simulink model "NarmaMotorNoDisrtubS2"  (R2019b)
settings: Solver=FixedStepAuto  StartTime=0.0  StopTime=30  FixedStep=0.001  RelTol=1e-3
libraries: neural x1, simulink x1
settings Model: Creator=Emanuel  LastModifiedBy=Emanuel

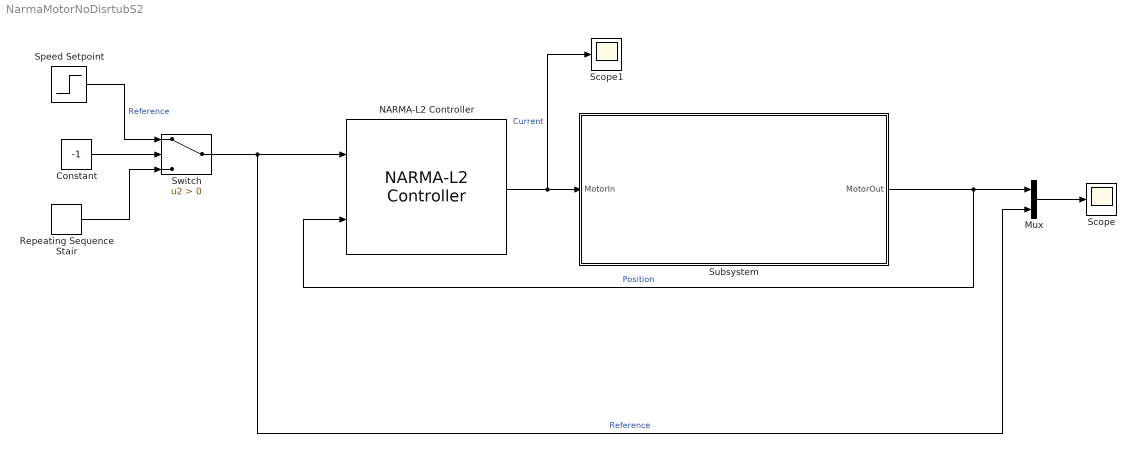
== system NarmaMotorNoDisrtubS2 ==
  Constant : Constant  Value=-1
  Mux : Mux  Inputs=2
  NARMA-L2 Controller : neural/Control Systems/NARMA-L2 Controller  Normalize=0  IW1_1=[-2.974276009383301389 -7.3369230181230387089 -2.9702809109209642457 5.4207339599484667403 7.6507322251574825245 -0.04099227858104749489 -7.6140400707472677411 6.5497336612263019617 4.8034287583779420316 4.8627156977741989863 4.9979580240842551575 12.428056540361712479 10.772508115065093648;-3.7848779205651705837 9.9348214966989338848 18.49827299409104242 -10.090455661305510304 -24.284030478949990339 -5.0384647207874486696 15.653492074662855416 -5.8472817958102094593 -8.3171263007948841306 -4.3483907391506937401 -4.3079358905802287438 -17.852109035411253046 -13.991455106924028939;2.4555196211613341539 -5.4285989222563859613 2.8335778045532187264 -2.2221660495332185015 -18.30929997074996507 0.9608078577356302663 19.398117488478394677 -3.5123739145945203077 -4.2568486454539327113 -5.5331001356038234107 -1.9069745865266656271 -13.104291606894983957 -10.684117094880070553;-15.725226773532602564 11.606034707360642244 -2.4238131705326448895 -10.051560874195246242 7.1499260224029228539 6.8182769946466530442 3.5300431413955801752 -11.667762420868049489 -9.1015914741785337583 -6.0904682598539059413 -14.082250724169222522 2.3580633500480736586 7.6612102121046756764;6.4288402912186972671 9.7333737129299500168 1.5125780634996242036 -4.4898243144994811615 -6.0240011150271524087 -6.203944305279691207 -6.7209811006371422692 9.0984885796634777932 9.6103820236549690748 10.946396320456580398 9.7071762450557628199 14.360221804286766201 13.530671886044359553;-0.00011769746202006098465 1.9131479129218529115e-05 2.1368830884739749535e-06 -2.2538716495860472075e-05 4.4301355498810600407e-05 -1.1306907536450035726e-05 -2.9413442925552235897e-06 -0.0002459300933314099275 0.00014022267822026942869 0.0001254313096875739103 -0.00010130255484437582073 7.0113646745459607193e-05 0.0002621578585166984914;-22.09980172382694974 22.698376943775290471 -14.547253951303501296 -2.1652344301828225781 8.2700319950257590307 5.8782840802360096788 0.47299538496945447985 -1.2446564177901784376 17.92268150488299483 12.162259495231486639 11.853079478572555061 19.970771843250901156 13.138667344604506582]  IW3_2=[1.706627376636813187 2.5735726820080659927 -6.1815669886082655893 0.57275147713232910096 -0.28158305950109818738 -0.40058963532887004177 2.0875189500048016988 -4.5176616794586568204 6.2034230229622489006 0.68314183246592163901 2.7222430817291480842 16.717543720164918852 4.2388903956459351718;10.854169291744398151 4.1599268772786528459 -0.9413361527648951288 -3.4661475675864905632 4.3656951082432797762 3.8319621471641625021 -19.907518954056317995 -13.190558582758342254 -1.7573075764144285849 -6.9276162312328413151 -9.971103171602539561 -18.488983191318666854 -12.655957966149603777;-0.074692547535554681959 0.12448824259257879055 -0.042378075841008985836 -0.0010633351392915922542 -0.047402972676021323806 0.0043997898900478707787 0.025542381717221347703 0.43643985176291932859 -0.040963191110162548714 -0.38753338727414143872 9.0232907589537507675 -4.6628698624088658065 -4.2513664191453219843;3.7161774522690635969 -2.5591393802404667213 -17.714639548587971518 -9.3452325709335468673 12.3521221043333842 18.349937714175496239 18.16388101440478664 -6.5735342650974502021 -1.9388343688512317264 -6.2028994712801530653 -6.9740804318796927319 -15.714806651937312409 -9.0848674503554676107;-0.38561792095397057212 -2.1655339591958520096 3.0795451086940848207 -3.5002169206264666101 -1.5721244517890888837 1.9118640186902990941 2.0413581201640433882 9.9227982049465719427 11.787525530972672527 19.775174712938209609 15.14987346971308213 57.285198652594829127 40.20055653107097271;1.4426181507754287647 -3.2930139520248609131 1.726100971075808399 0.19760804767428463702 -2.7092348185502794777 0.32884589914935780097 2.0362016858337690373 10.354919037811358251 -3.6494508377007615074 12.170550474039952604 1.0545829836571187776 32.166978404432839511 47.464270694044230936;2.1106579591855849642 2.3628910055998768591 -1.7320235272860964315 -1.7164755498128061451 0.21780801521552364819 0.5013567452443652428 -3.2326650559587317701 -0.54820111612144706292 -0.58988404458119769735 -0.18463996511002475631 -0.29562382702827300074 1.3704222651936768251 2.1199608105666714053]  IW5_3=0.042885061780776181917  LW2_1=[-1.7951544843657809558 -0.77607352941402596436 0.028588755459878215787 -0.19678846492423079928 -51.119414104473214877 -178.5855067132064562 -0.066423346363697524652]  LW4_3=[0.63499890113034485051 -1.1080571969744621441 -6.7043348300094498526 3.8041307269777782096 1.5163618754587511184 -1.5268705266003823606 -9.054353426704784269]  LW5_4=3.1544506198367718852  LW6_5=1.8181754716409308514  LW6_2=63.390639269687206081  B1=[0.80241417086431465755;2.1611243877218009324;-1.6799171806335817525;-3.3987486888518860795;-2.9163481938314257391;0.60217891806372336738;-3.2240787265158776798]  B2=53.798959508292931275  B3=[-3.3581424805022304092;-0.021276709706567312891;41.425727380152643775;-0.041722817605074846714;-1.6885845638705636595;-46.221330514506583143;-0.42269984660533566068]  B4=6.1467763144405829223  Limit_output=0  min_output=-Inf  max_output=Inf  Use_Previous_Weights=1  Ts=0.05  S1=7  Ni=7  Nj=7  sim_file=SoleModelNoDistrubance  trainfun=trainlm  Use_validation=1  Use_Testing=1  max_i=40  min_i=1  max_i_int=4  min_i_int=2  sam_training=10000  epochs=500  minp=1.2838861864609374397  maxp=39.753006491435613157  mint=2000.3866487334141766  maxt=39.753006491435613157
      settings: SourceProductName=Deep Learning Toolbox  SourceProductBaseCode=NN
  Repeating Sequence Stair : simulink/Sources/Repeating Sequence Stair  OutValues=[1000 2000 3000 4000 5000].'  tsamp=4  OutMin=[]  OutMax=[]  OutDataTypeStr=double  OutputDataTypeScalingMode=double  OutDataType=fixdt(0,8)  ConRadixGroup=Best Precision: Vector-wise  OutScaling=2^-12
  Scope : Scope
  Scope1 : Scope
  Speed Setpoint : Step  Time=5  Before=2000  After=3000  SampleTime=0
  Subsystem : Subsystem
  Switch : Switch  Criteria=u2 > Threshold
  wires:
  NARMA-L2 Controller/1 -> Scope1/1, Subsystem/1(MotorIn)  "Current"
  Subsystem/1("MotorOut ") -> NARMA-L2 Controller/2, Mux/1  "Position"
  Mux/1 -> Scope/1
  Switch/1 -> Mux/2, NARMA-L2 Controller/1  "Reference"
  Repeating Sequence Stair/1 -> Switch/3
  Speed Setpoint/1 -> Switch/1  "Reference"
  Constant/1 -> Switch/2

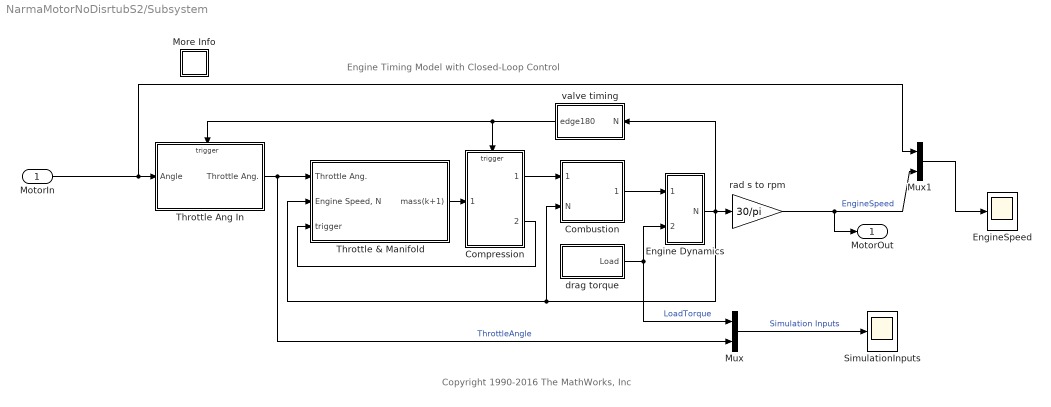
== system NarmaMotorNoDisrtubS2/Subsystem ==
  note: Copyright 1990-2016 The MathWorks, Inc
  note: Engine Timing Model with Closed-Loop Control
  MotorIn : Inport
  Combustion : Subsystem
  Compression : Subsystem  TreatAsAtomicUnit=on
  Engine Dynamics : Subsystem
  EngineSpeed : Scope
  More Info : Subsystem
      settings: OpenFcn=showdemo(bdroot(gcb))
      mask Display: disp('?')
  Mux : Mux  Inputs=2
  Mux1 : Mux  Inputs=2
  SimulationInputs : Scope
  Throttle & Manifold : Subsystem
  Throttle Ang In : Subsystem  TreatAsAtomicUnit=on
  drag torque : Subsystem
  rad s to rpm : Gain  Gain=30/pi  SaturateOnIntegerOverflow=on  OutDataTypeStr=Inherit: Same as input  ParamDataTypeStr=Inherit: Same as input
  valve timing : Subsystem
  "MotorOut " : Outport
  wires:
  Combustion/1(Torque) -> Engine Dynamics/1(Teng)
  Throttle Ang In/1(Throttle Ang.) -> Mux/2, Throttle & Manifold/1(Throttle Ang.)  "ThrottleAngle"
  drag torque/1(Load) -> Mux/1, Engine Dynamics/2(Tload)  "LoadTorque"
  MotorIn/1 -> Mux1/1, Throttle Ang In/1(Angle)
  Throttle & Manifold/1(mass(k+1)) -> Compression/1(mass(k+1))
  Compression/2(trigger) -> Throttle & Manifold/3(trigger)
  Mux/1 -> SimulationInputs/1  "Simulation Inputs"
  rad s to rpm/1 -> "MotorOut "/1, Mux1/2  "EngineSpeed"
  Compression/1(mass(k)) -> Combustion/1(Air Charge)
  Mux1/1 -> EngineSpeed/1
  valve timing/1(edge180) -> Throttle Ang In/Trigger, Compression/Trigger
  Engine Dynamics/1(N) -> rad s to rpm/1, valve timing/1(N), Throttle & Manifold/2("Engine Speed, N"), Combustion/2(N)

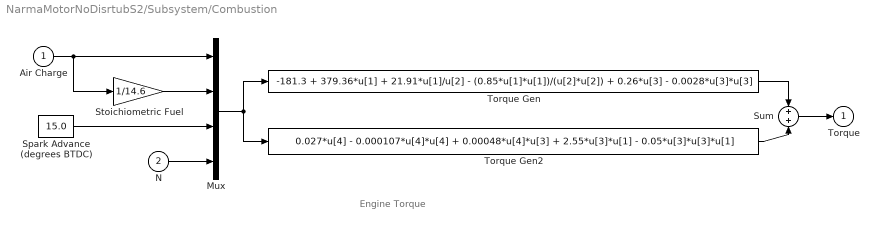
== system NarmaMotorNoDisrtubS2/Subsystem/Combustion ==
  note: Engine Torque
  Air Charge : Inport
  N : Inport  Port=2
  Mux : Mux
  Spark Advance (degrees BTDC) : Constant  Value=15.0
  Stoichiometric Fuel : Gain  Gain=1/14.6  SaturateOnIntegerOverflow=on  OutDataTypeStr=Inherit: Same as input  ParamDataTypeStr=Inherit: Same as input
  Sum : Sum  SaturateOnIntegerOverflow=on  InputSameDT=on  OutDataTypeStr=Inherit: Same as first input
  Torque Gen : Fcn  Expr=-181.3 + 379.36*u[1] + 21.91*u[1]/u[2] - (0.85*u[1]*u[1])/(u[2]*u[2]) + 0.26*u[3] - 0.0028*u[3]*u[3]
  Torque Gen2 : Fcn  Expr=0.027*u[4] - 0.000107*u[4]*u[4] + 0.00048*u[4]*u[3] + 2.55*u[3]*u[1] - 0.05*u[3]*u[3]*u[1]
  Torque : Outport  InitialOutput=0
  wires:
  Stoichiometric Fuel/1 -> Mux/2
  Spark Advance (degrees BTDC)/1 -> Mux/3
  N/1 -> Mux/4
  Air Charge/1 -> Stoichiometric Fuel/1, Mux/1
  Mux/1 -> Torque Gen/1, Torque Gen2/1
  Torque Gen2/1 -> Sum/2
  Torque Gen/1 -> Sum/1
  Sum/1 -> Torque/1

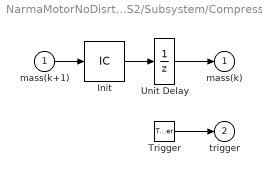
== system NarmaMotorNoDisrtubS2/Subsystem/Compression ==
  mass(k+1) : Inport
  Trigger : TriggerPort  TriggerType=either  VariantControl=Variant  ShowOutputPort=on
  Init : InitialCondition  Value=0.152
  Unit Delay : UnitDelay  InitialCondition=0.152  SampleTime=-1  HasFrameUpgradeWarning=on
  mass(k) : Outport  InitialOutput=0.152
  trigger : Outport  Port=2  InitialOutput=-1
  wires:
  Init/1 -> Unit Delay/1
  mass(k+1)/1 -> Init/1
  Unit Delay/1 -> mass(k)/1
  Trigger/1 -> trigger/1

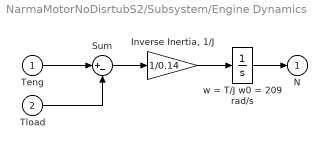
== system NarmaMotorNoDisrtubS2/Subsystem/Engine Dynamics ==
  Teng : Inport
  Tload : Inport  Port=2
  "Inverse Inertia, 1/J" : Gain  Gain=1/0.14  SaturateOnIntegerOverflow=on  OutDataTypeStr=Inherit: Same as input  ParamDataTypeStr=Inherit: Same as input
  Sum : Sum  Inputs=|+-  SaturateOnIntegerOverflow=on  InputSameDT=on  OutDataTypeStr=Inherit: Same as first input
  w = T/J w0 = 209 rad/s : Integrator  InitialCondition=209.48
  N : Outport  InitialOutput=0
  wires:
  "Inverse Inertia, 1/J"/1 -> w = T/J w0 = 209 rad/s/1
  w = T/J w0 = 209 rad/s/1 -> N/1
  Sum/1 -> "Inverse Inertia, 1/J"/1
  Teng/1 -> Sum/1
  Tload/1 -> Sum/2

== system NarmaMotorNoDisrtubS2/Subsystem/More Info ==

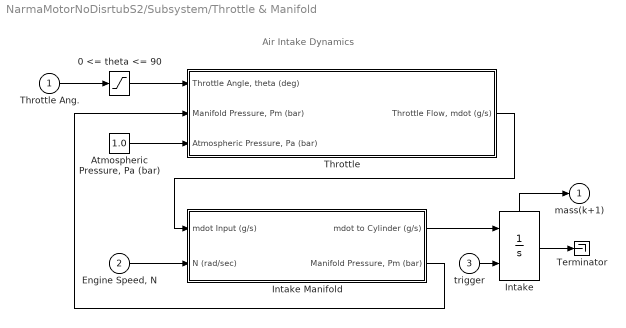
== system NarmaMotorNoDisrtubS2/Subsystem/Throttle & Manifold ==
  note: Air Intake Dynamics
  Throttle Ang. : Inport
  "Engine Speed, N" : Inport  Port=2
  trigger : Inport  Port=3
  0 <= theta <= 90 : Saturate  UpperLimit=90  LowerLimit=0
  "Atmospheric Pressure, Pa (bar)" : Constant  Value=1.0
  Intake : Integrator  ExternalReset=either  ShowStatePort=on
  Intake Manifold : Subsystem
  Terminator : Terminator
  Throttle : Subsystem
  mass(k+1) : Outport  InitialOutput=0
  wires:
  0 <= theta <= 90/1 -> Throttle/1("Throttle Angle, theta (deg)")
  Throttle Ang./1 -> 0 <= theta <= 90/1
  Throttle/1("Throttle Flow, mdot (g/s)") -> Intake Manifold/1(mdot Input (g/s))
  "Engine Speed, N"/1 -> Intake Manifold/2(N (rad/sec))
  Intake Manifold/2("Manifold Pressure, Pm (bar)") -> Throttle/2("Manifold Pressure, Pm (bar)")
  Intake Manifold/1(mdot to Cylinder (g/s)) -> Intake/1
  "Atmospheric Pressure, Pa (bar)"/1 -> Throttle/3("Atmospheric Pressure, Pa (bar) ")
  Intake/State -> mass(k+1)/1
  trigger/1 -> Intake/2
  Intake/1 -> Terminator/1

== system NarmaMotorNoDisrtubS2/Subsystem/Throttle Ang In ==
  note: Controller Subsystem
  Angle : Inport
  Trigger : TriggerPort  TriggerType=either  VariantControl=Variant
  Throttle Ang. : Outport  InitialOutput=8.973
  wires:
  Angle/1 -> Throttle Ang./1

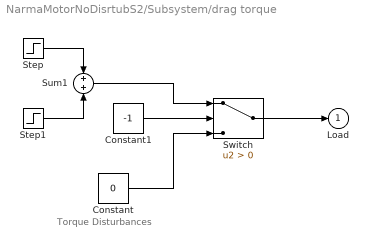
== system NarmaMotorNoDisrtubS2/Subsystem/drag torque ==
  note: Torque Disturbances
  Constant : Constant  Value=0
  Constant1 : Constant  Value=-1
  Step : Step  Time=2  Before=25  After=20  SampleTime=0
  Step1 : Step  Time=8  After=5  SampleTime=0
  Sum1 : Sum  SaturateOnIntegerOverflow=on  InputSameDT=on  OutDataTypeStr=Inherit: Same as first input
  Switch : Switch  Criteria=u2 > Threshold
  Load : Outport  InitialOutput=0
  wires:
  Sum1/1 -> Switch/1
  Step/1 -> Sum1/1
  Step1/1 -> Sum1/2
  Switch/1 -> Load/1
  Constant/1 -> Switch/3
  Constant1/1 -> Switch/2

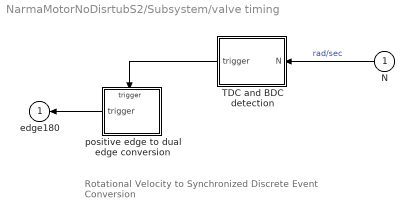
== system NarmaMotorNoDisrtubS2/Subsystem/valve timing ==
  note: Rotational Velocity to Synchronized
      | Discrete Event Conversion
  N : Inport
  TDC and BDC detection : Subsystem
  positive edge to dual edge conversion : Subsystem  TreatAsAtomicUnit=on
  edge180 : Outport  InitialOutput=-1
  wires:
  TDC and BDC detection/1(trigger) -> positive edge to dual edge conversion/Trigger
  positive edge to dual edge conversion/1(trigger) -> edge180/1
  N/1 -> TDC and BDC detection/1(N)  "rad/sec"

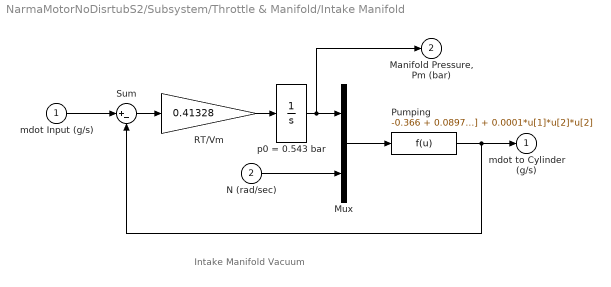
== system NarmaMotorNoDisrtubS2/Subsystem/Throttle & Manifold/Intake Manifold ==
  note: Intake Manifold Vacuum
  mdot Input (g/s) : Inport
  N (rad/sec) : Inport  Port=2
  Mux : Mux  Inputs=2
  Pumping : Fcn  Expr=-0.366 + 0.08979*u[1]*u[2] - 0.0337*u[2]*u[1]*u[1] + 0.0001*u[1]*u[2]*u[2]
  RT/Vm : Gain  Gain=0.41328  SaturateOnIntegerOverflow=on  OutDataTypeStr=Inherit: Same as input  ParamDataTypeStr=Inherit: Same as input
  Sum : Sum  Inputs=|+-  SaturateOnIntegerOverflow=on  InputSameDT=on  OutDataTypeStr=Inherit: Same as first input
  p0 = 0.543 bar : Integrator  InitialCondition=.543
  mdot to Cylinder (g/s) : Outport  InitialOutput=0
  "Manifold Pressure, Pm (bar)" : Outport  Port=2  InitialOutput=0
  wires:
  mdot Input (g/s)/1 -> Sum/1
  RT/Vm/1 -> p0 = 0.543 bar/1
  N (rad/sec)/1 -> Mux/2
  Mux/1 -> Pumping/1
  p0 = 0.543 bar/1 -> Mux/1, "Manifold Pressure, Pm (bar)"/1
  Sum/1 -> RT/Vm/1
  Pumping/1 -> Sum/2, mdot to Cylinder (g/s)/1

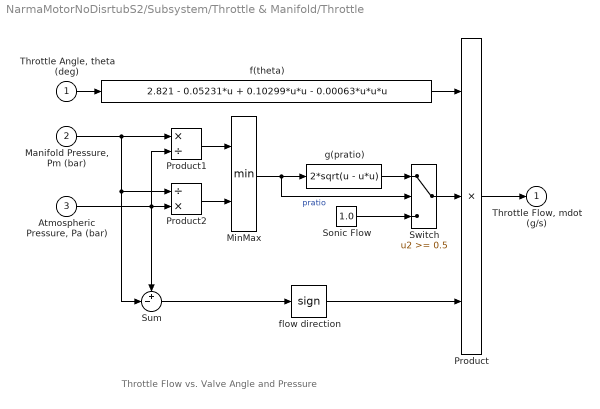
== system NarmaMotorNoDisrtubS2/Subsystem/Throttle & Manifold/Throttle ==
  note: Throttle Flow vs. Valve Angle and Pressure
  "Throttle Angle, theta (deg)" : Inport
  "Manifold Pressure, Pm (bar)" : Inport  Port=2
  "Atmospheric Pressure, Pa (bar) " : Inport  Port=3
  MinMax : MinMax  Inputs=2  SaturateOnIntegerOverflow=on  InputSameDT=on
  Product : Product  Inputs=3  SaturateOnIntegerOverflow=on  RndMeth=Zero  InputSameDT=on  OutDataTypeStr=Inherit: Same as first input
  Product1 : Product  Inputs=*/  SaturateOnIntegerOverflow=on  RndMeth=Zero  InputSameDT=on  OutDataTypeStr=Inherit: Same as first input
  Product2 : Product  Inputs=/*  SaturateOnIntegerOverflow=on  RndMeth=Zero  InputSameDT=on  OutDataTypeStr=Inherit: Same as first input
  "Sonic Flow " : Constant  Value=1.0
  Sum : Sum  Inputs=+-|  SaturateOnIntegerOverflow=on  InputSameDT=on  OutDataTypeStr=Inherit: Same as first input
  Switch : Switch  Threshold=0.5  SaturateOnIntegerOverflow=on  InputSameDT=on
  f(theta) : Fcn  Expr=2.821 - 0.05231*u + 0.10299*u*u - 0.00063*u*u*u
  flow direction : Signum
  g(pratio) : Fcn  Expr=2*sqrt(u - u*u)
  "Throttle Flow, mdot (g/s)" : Outport  InitialOutput=0
  wires:
  "Manifold Pressure, Pm (bar)"/1 -> Sum/2, Product2/1, Product1/1
  Product2/1 -> MinMax/2
  Product1/1 -> MinMax/1
  "Atmospheric Pressure, Pa (bar) "/1 -> Sum/1, Product2/2, Product1/2
  g(pratio)/1 -> Switch/1
  "Sonic Flow "/1 -> Switch/3
  Switch/1 -> Product/2
  flow direction/1 -> Product/3
  Sum/1 -> flow direction/1
  MinMax/1 -> Switch/2, g(pratio)/1  "pratio"
  "Throttle Angle, theta (deg)"/1 -> f(theta)/1
  Product/1 -> "Throttle Flow, mdot (g/s)"/1
  f(theta)/1 -> Product/1

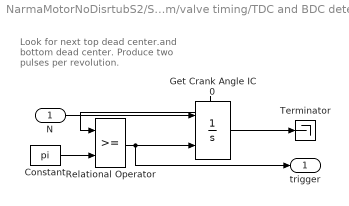
== system NarmaMotorNoDisrtubS2/Subsystem/valve timing/TDC and BDC detection ==
  note: Look for next top dead center.and
      | bottom dead center.
      | Produce two pulses per revolution.
  N : Inport
  Constant : Constant  Value=pi
  Get Crank Angle IC 0 : Integrator  ExternalReset=rising  ShowStatePort=on
  Relational Operator : RelationalOperator  OutDataTypeStr=boolean  RndMeth=Nearest  InputSameDT=on
  Terminator : Terminator
  trigger : Outport  InitialOutput=0
  wires:
  N/1 -> Get Crank Angle IC 0/1
  Relational Operator/1 -> trigger/1, Get Crank Angle IC 0/2
  Constant/1 -> Relational Operator/2
  Get Crank Angle IC 0/State -> Relational Operator/1
  Get Crank Angle IC 0/1 -> Terminator/1

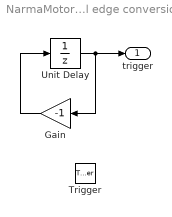
== system NarmaMotorNoDisrtubS2/Subsystem/valve timing/positive edge to dual edge conversion ==
  Trigger : TriggerPort  VariantControl=Variant
  Gain : Gain  Gain=-1  SaturateOnIntegerOverflow=on  OutDataTypeStr=Inherit: Same as input  ParamDataTypeStr=Inherit: Same as input
  Unit Delay : UnitDelay  InitialCondition=1  SampleTime=-1  HasFrameUpgradeWarning=on
  trigger : Outport  InitialOutput=-1
  wires:
  Gain/1 -> Unit Delay/1
  Unit Delay/1 -> trigger/1, Gain/1
